simulink model "Linearize_Bare_Airframe"  (R2022a)
settings: Solver=VariableStepAuto  StartTime=0.0  StopTime=10.0  RelTol=1e-3
undefined symbols (not defined in the file): Aactuator, ac, AeroCoeff, EngineTable, F, fs, ft, g, hground, IC, kg, LandingGear, Light, m, MIL, s, Sensor, slug, state0, WMM2020
libraries: aerolibconvert2 x15, simulink x4, aerolibatmos2 x3, aerolibwind2 x3, sharedutil x3, aerolibbdyn x3, aerolibgravity2 x2, sharedtransform x1
(part 2 of 4)

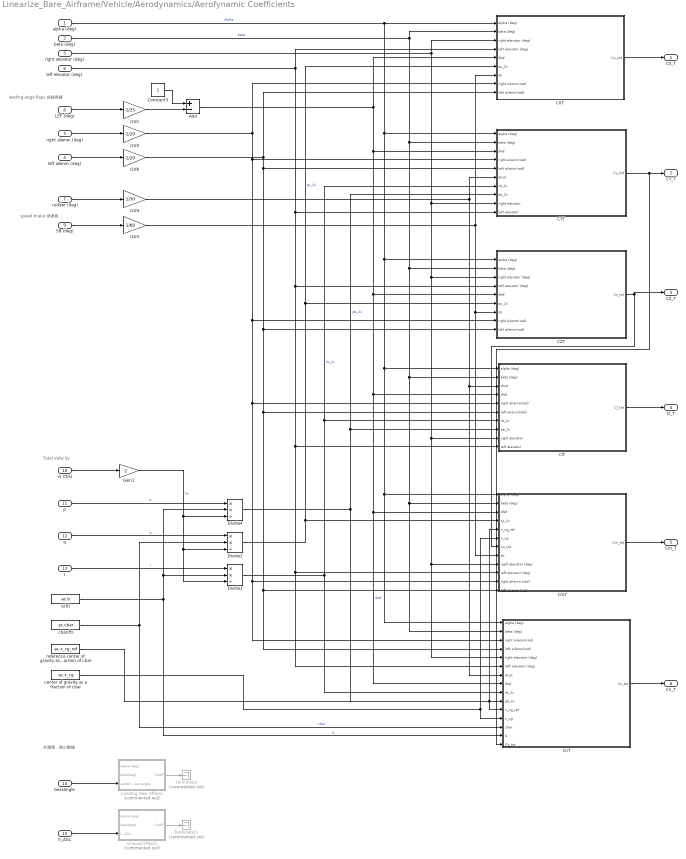
== system Linearize_Bare_Airframe/Vehicle/Aerodynamics/Aerofynamic Coefficients ==
  note: Total Velocity
  note: 未建模，缺少數據
  note: speed brake
      | 減速板
  note: leading-edge flaps
      | 前緣襟翼
  alpha (deg) : Inport
  beta (deg) : Inport  Port=2
  right alieron (deg) : Inport  Port=3
  left aileron (deg) : Inport  Port=4
  right elevator (deg) : Inport  Port=5
  left elevator (deg) : Inport  Port=6
  rudder (deg) : Inport  Port=7
  LEF (deg) : Inport  Port=8
  SB (deg) : Inport  Port=9
  vt (ft/s) : Inport  Port=10
  p : Inport  Port=11
  q : Inport  Port=12
  r : Inport  Port=13
  GearAngle : Inport  Port=14
  h_AGL : Inport  Port=15
  Add : Sum  Inputs=+-
  CXT : Subsystem
  CYT : Subsystem
  CZT : Subsystem
  ClT : Subsystem
  CmT : Subsystem
  CnT : Subsystem
  Constant3 : Constant
  Divide2 : Product  Inputs=**/
  Divide3 : Product  Inputs=**/
  Divide4 : Product  Inputs=**/
  Gain1 : Gain  Gain=2
  Ground Effects : Subsystem  Commented=on
  Landing Gear Effects : Subsystem  Commented=on
  Terminator : Terminator  Commented=on
  Terminator1 : Terminator  Commented=on
  b(ft) : Constant  Value=ac.b
  cbar(ft) : Constant  Value=ac.cbar
  center of gravity as a fraction of cbar : Constant  Value=ac.x_cg
  r2d1 : Gain  Gain=1/25  SaturateOnIntegerOverflow=on  OutDataTypeStr=Inherit: Same as input  ParamDataTypeStr=Inherit: Same as input
  r2d3 : Gain  Gain=1/60  SaturateOnIntegerOverflow=on  OutDataTypeStr=Inherit: Same as input  ParamDataTypeStr=Inherit: Same as input
  r2d4 : Gain  Gain=1/30  SaturateOnIntegerOverflow=on  OutDataTypeStr=Inherit: Same as input  ParamDataTypeStr=Inherit: Same as input
  r2d5 : Gain  Gain=1/20  SaturateOnIntegerOverflow=on  OutDataTypeStr=Inherit: Same as input  ParamDataTypeStr=Inherit: Same as input
  r2d6 : Gain  Gain=1/20  SaturateOnIntegerOverflow=on  OutDataTypeStr=Inherit: Same as input  ParamDataTypeStr=Inherit: Same as input
  reference center of gravity as a fraction of cbar : Constant  Value=ac.x_cg_ref
  CX_T : Outport  VectorParamsAs1DForOutWhenUnconnected=off
  CY_T : Outport  Port=2  VectorParamsAs1DForOutWhenUnconnected=off
  CZ_T : Outport  Port=3  VectorParamsAs1DForOutWhenUnconnected=off
  Cl_T : Outport  Port=4  VectorParamsAs1DForOutWhenUnconnected=off
  Cm_T : Outport  Port=5  VectorParamsAs1DForOutWhenUnconnected=off
  Cn_T : Outport  Port=6  VectorParamsAs1DForOutWhenUnconnected=off
  wires:
  alpha (deg)/1 -> CnT/1(alpha (deg)), CmT/1(alpha (deg)), ClT/1(alpha (deg)), CZT/1(alpha (deg)), CYT/1(alpha (deg)), CXT/1(alpha (deg))  "alpha"
  beta (deg)/1 -> CnT/2(beta (deg)), CmT/2(beta (deg)), ClT/2(beta (deg)), CZT/2(beta (deg)), CYT/2(beta (deg)), CXT/2("beta (deg) ")  "beta"
  right elevator (deg)/1 -> CmT/9(right elevator (deg)), CnT/5("right elevator (deg) "), ClT/9(right elevator), CZT/3(right elevator (deg)), CYT/9(right elevator), CXT/3(right elevator (deg))
  vt (ft/s)/1 -> Gain1/1
  q/1 -> Divide2/1  "q"
  r/1 -> Divide3/1  "r"
  Divide2/1 -> CXT/6(qc_2v), CZT/6(qc_2v), CmT/4(qc_2v)  "qc_2v"
  Divide3/1 -> CYT/7(rb_2v), ClT/7(rb_2v), CnT/9(rb_2v)  "rb_2v"
  Divide4/1 -> CYT/8(pb_2v), ClT/8(pb_2v), CnT/10(pb_2v)  "pb_2v"
  b(ft)/1 -> CnT/14(b), Divide3/2, Divide4/2  "b"
  cbar(ft)/1 -> CnT/13(cbar), Divide2/2  "cbar"
  reference center of gravity as a fraction of cbar/1 -> CmT/5(x_cg_ref), CnT/11(x_cg_ref)
  center of gravity as a fraction of cbar/1 -> CmT/6(x_cg), CnT/12(x_cg)
  CZT/1(Cz_tot) -> CZ_T/1, CmT/7(Cz_tot)
  CYT/1(Cy_tot) -> CnT/15(Cy_tot), CY_T/1
  CXT/1(Cx_tot) -> CX_T/1
  ClT/1(Cl_tot) -> Cl_T/1
  CmT/1(Cm_tot) -> Cm_T/1
  CnT/1(Cn_tot) -> Cn_T/1
  Add/1 -> CXT/5(dlef), CnT/8(dlef), CmT/3(dlef), ClT/4(dlef), CZT/5(dlef), CYT/3(dlef)  "dlef"
  rudder (deg)/1 -> r2d4/1
  SB (deg)/1 -> r2d3/1
  r2d1/1 -> Add/2
  Constant3/1 -> Add/1
  LEF (deg)/1 -> r2d1/1
  Gain1/1 -> Divide4/3, Divide3/3, Divide2/3  "2v"
  p/1 -> Divide4/1  "p"
  r2d3/1 -> CmT/8(sb), CZT/7(sb), CXT/7(sb)
  r2d4/1 -> CYT/6(drud), CnT/7(drud), ClT/3(drud)
  GearAngle/1 -> Landing Gear Effects/3(Landing Gear Angle)
  h_AGL/1 -> Ground Effects/3(h_AGL)
  Landing Gear Effects/1(Coeff) -> Terminator/1
  Ground Effects/1(Coeff) -> Terminator1/1
  left elevator (deg)/1 -> CZT/4(left elevator (deg)), CmT/10(left elevator (deg)), CnT/6(left elevator (deg)), ClT/10(left elevator), CYT/10(left elevator), CXT/4(left elevator (deg))
  right alieron (deg)/1 -> r2d5/1
  left aileron (deg)/1 -> r2d6/1
  r2d5/1 -> CmT/11(right aileron (rad)), CnT/3(right aileron(rad)), ClT/5(right aileron(rad)), CZT/8(right aileron(rad)), CYT/4(right aileron(rad)), CXT/8(right aileron(rad))
  r2d6/1 -> CXT/9(left aileron(rad)), CZT/9(left aileron(rad)), CmT/12(left aileron (rad)), CnT/4(left aileron(rad)), ClT/6(left aileron(rad)), CYT/5(left aileron(rad))

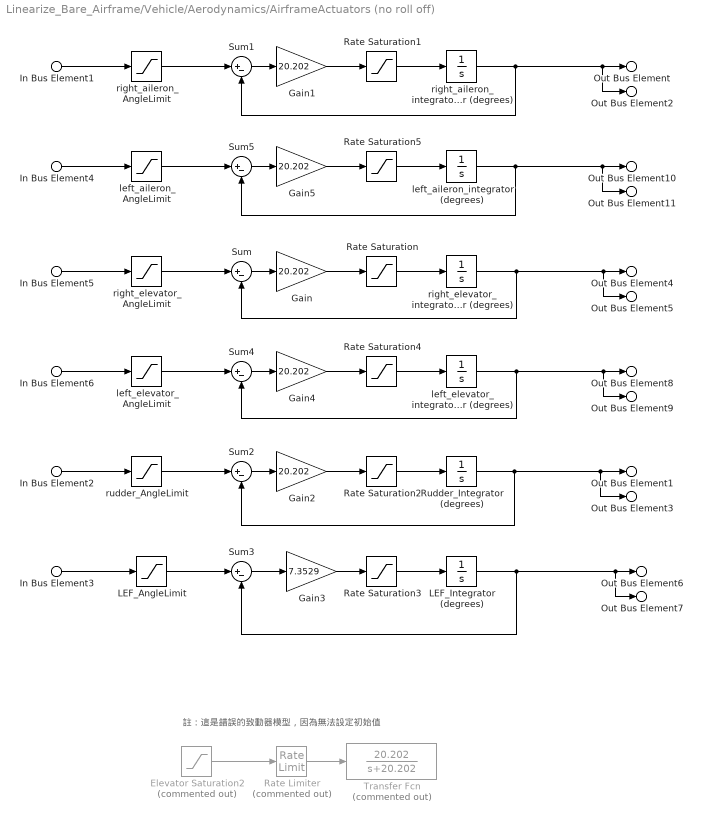
== system Linearize_Bare_Airframe/Vehicle/Aerodynamics/AirframeActuators (no roll off) ==
  note: 註：這是錯誤的致動器模型，因為無法設定初始值
  In Bus Element2 : Inport  PortName=fcs_cmd  Element=rudder
  In Bus Element3 : Inport  PortName=fcs_cmd  Element=LEF
  In Bus Element4 : Inport  PortName=fcs_cmd  Element=left aileron
  In Bus Element5 : Inport  PortName=fcs_cmd  Element=right elevator
  In Bus Element6 : Inport  PortName=fcs_cmd  Element=left elevator
  In Bus Element1 : Inport  PortName=fcs_cmd  Element=right aileron
  Elevator Saturation2 : Saturate  Commented=on  UpperLimit=25  LowerLimit=-25
  Gain{,1..2,4..5} (5 alike) : Gain  Gain=20.202  SaturateOnIntegerOverflow=on  OutDataTypeStr=Inherit: Same as input  ParamDataTypeStr=Inherit: Same as input
  Gain3 : Gain  Gain=7.3529  SaturateOnIntegerOverflow=on  OutDataTypeStr=Inherit: Same as input  ParamDataTypeStr=Inherit: Same as input
  LEF_AngleLimit : Saturate  UpperLimit=Aactuator.LEF.AngleLimitUpper  LowerLimit=Aactuator.LEF.AngleLimitLower
  LEF_Integrator (degrees) : Integrator  InitialCondition=Aactuator.LEF.IntegratorInitial  LimitOutput=on  UpperSaturationLimit=Aactuator.LEF.AngleLimitUpper  LowerSaturationLimit=Aactuator.LEF.AngleLimitLower
  Rate Saturation : Saturate  UpperLimit=Aactuator.right_elevator.RateLimitUpper  LowerLimit=Aactuator.right_elevator.RateLimitLower
  Rate Saturation1 : Saturate  UpperLimit=Aactuator.right_aileron.RateLimitUpper  LowerLimit=Aactuator.right_aileron.RateLimitLower
  Rate Saturation2 : Saturate  UpperLimit=Aactuator.rudder.RateLimitUpper  LowerLimit=Aactuator.rudder.RateLimitLower
  Rate Saturation3 : Saturate  UpperLimit=Aactuator.LEF.RateLimitUpper  LowerLimit=Aactuator.LEF.RateLimitLower
  Rate Saturation4 : Saturate  UpperLimit=Aactuator.left_elevator.RateLimitUpper  LowerLimit=Aactuator.left_elevator.RateLimitLower
  Rate Saturation5 : Saturate  UpperLimit=Aactuator.left_aileron.RateLimitUpper  LowerLimit=Aactuator.left_aileron.RateLimitLower
  Rate Limiter : RateLimiter  Commented=on  RisingSlewLimit=+60  FallingSlewLimit=-60  SampleTimeMode=inherited
  Rudder_Integrator (degrees) : Integrator  InitialCondition=Aactuator.rudder.IntegratorInitial  LimitOutput=on  UpperSaturationLimit=Aactuator.rudder.AngleLimitUpper  LowerSaturationLimit=Aactuator.rudder.AngleLimitLower
  Sum{,1..5} (6 alike) : Sum  Inputs=|+-  InputSameDT=on  SaturateOnIntegerOverflow=on  OutDataTypeStr=Inherit: Same as first input
  Transfer Fcn : TransferFcn  Commented=on  Numerator=[20.202]  Denominator=[1 20.202]
  left_aileron_AngleLimit : Saturate  UpperLimit=Aactuator.left_aileron.AngleLimitUpper  LowerLimit=Aactuator.left_aileron.AngleLimitLower
  left_aileron_integrator (degrees) : Integrator  InitialCondition=Aactuator.left_aileron.IntegratorInitial  LimitOutput=on  UpperSaturationLimit=Aactuator.left_aileron.AngleLimitUpper  LowerSaturationLimit=Aactuator.left_aileron.AngleLimitLower
  left_elevator_AngleLimit : Saturate  UpperLimit=Aactuator.left_elevator.AngleLimitUpper  LowerLimit=Aactuator.left_elevator.AngleLimitLower
  left_elevator_integrator (degrees) : Integrator  InitialCondition=Aactuator.left_elevator.IntegratorInitial  LimitOutput=on  UpperSaturationLimit=Aactuator.left_elevator.AngleLimitUpper  LowerSaturationLimit=Aactuator.left_elevator.AngleLimitLower
  right_aileron_AngleLimit : Saturate  UpperLimit=Aactuator.right_aileron.AngleLimitUpper  LowerLimit=Aactuator.right_aileron.AngleLimitLower
  right_aileron_integrator (degrees) : Integrator  InitialCondition=Aactuator.right_aileron.IntegratorInitial  LimitOutput=on  UpperSaturationLimit=Aactuator.right_aileron.AngleLimitUpper  LowerSaturationLimit=Aactuator.right_aileron.AngleLimitLower
  right_elevator_AngleLimit : Saturate  UpperLimit=Aactuator.right_elevator.AngleLimitUpper  LowerLimit=Aactuator.right_elevator.AngleLimitLower  LinearizeAsGain=off
  right_elevator_integrator (degrees) : Integrator  InitialCondition=Aactuator.right_elevator.IntegratorInitial  LimitOutput=on  UpperSaturationLimit=Aactuator.right_elevator.AngleLimitUpper  LowerSaturationLimit=Aactuator.right_elevator.AngleLimitLower
  rudder_AngleLimit : Saturate  UpperLimit=Aactuator.rudder.AngleLimitUpper  LowerLimit=Aactuator.rudder.AngleLimitLower
  Out Bus Element : Outport  PortName=ActPositions  Element=right Aileron_deg
  Out Bus Element1 : Outport  PortName=ActPositions  Element=Rudder_deg
  Out Bus Element4 : Outport  PortName=ActPositions  Element=right Elevator_deg
  Out Bus Element6 : Outport  PortName=ActPositions  Element=LEF_deg
  Out Bus Element8 : Outport  PortName=ActPositions  Element=left Elevator_deg
  Out Bus Element10 : Outport  PortName=ActPositions  Element=left Aileron_deg
  Out Bus Element2 : Outport  Port=2  PortName=ActSensor_Out  Element=right Aileron_deg
  Out Bus Element3 : Outport  Port=2  PortName=ActSensor_Out  Element=Rudder_deg
  Out Bus Element5 : Outport  Port=2  PortName=ActSensor_Out  Element=right Elevator_deg
  Out Bus Element7 : Outport  Port=2  PortName=ActSensor_Out  Element=LEF_deg
  Out Bus Element9 : Outport  Port=2  PortName=ActSensor_Out  Element=left Elevator_deg
  Out Bus Element11 : Outport  Port=2  PortName=ActSensor_Out  Element=left Aileron_deg
  wires:
  Gain/1 -> Rate Saturation/1
  Gain1/1 -> Rate Saturation1/1
  In Bus Element5/1 -> right_elevator_AngleLimit/1
  Rate Saturation/1 -> right_elevator_integrator (degrees)/1
  right_aileron_integrator (degrees)/1 -> Out Bus Element2/1, Out Bus Element/1, Sum1/2
  Rate Saturation1/1 -> right_aileron_integrator (degrees)/1
  Gain2/1 -> Rate Saturation2/1
  Sum1/1 -> Gain1/1
  Rudder_Integrator (degrees)/1 -> Out Bus Element3/1, Out Bus Element1/1, Sum2/2
  Rate Saturation2/1 -> Rudder_Integrator (degrees)/1
  Sum/1 -> Gain/1
  Sum2/1 -> Gain2/1
  right_elevator_integrator (degrees)/1 -> Sum/2, Out Bus Element5/1, Out Bus Element4/1
  In Bus Element1/1 -> right_aileron_AngleLimit/1
  In Bus Element2/1 -> rudder_AngleLimit/1
  LEF_Integrator (degrees)/1 -> Out Bus Element6/1, Out Bus Element7/1, Sum3/2
  In Bus Element3/1 -> LEF_AngleLimit/1
  Sum3/1 -> Gain3/1
  Rate Saturation3/1 -> LEF_Integrator (degrees)/1
  Gain3/1 -> Rate Saturation3/1
  Sum4/1 -> Gain4/1
  Gain4/1 -> Rate Saturation4/1
  Rate Saturation4/1 -> left_elevator_integrator (degrees)/1
  In Bus Element6/1 -> left_elevator_AngleLimit/1
  left_elevator_integrator (degrees)/1 -> Sum4/2, Out Bus Element9/1, Out Bus Element8/1
  Gain5/1 -> Rate Saturation5/1
  Rate Saturation5/1 -> left_aileron_integrator (degrees)/1
  Sum5/1 -> Gain5/1
  left_aileron_integrator (degrees)/1 -> Out Bus Element11/1, Out Bus Element10/1, Sum5/2
  In Bus Element4/1 -> left_aileron_AngleLimit/1
  right_aileron_AngleLimit/1 -> Sum1/1
  left_aileron_AngleLimit/1 -> Sum5/1
  left_elevator_AngleLimit/1 -> Sum4/1
  right_elevator_AngleLimit/1 -> Sum/1
  rudder_AngleLimit/1 -> Sum2/1
  LEF_AngleLimit/1 -> Sum3/1
  Rate Limiter/1 -> Transfer Fcn/1
  Elevator Saturation2/1 -> Rate Limiter/1

== system Linearize_Bare_Airframe/Vehicle/Aerodynamics/Leading Edge Flap ==
  note: $\delta_{LEF} =1.38\frac{2s+7.25}{s+7.25}\alpha -9.05\frac{\bar{q} }{p_s }+1.45$
      | $\alpha$ 的單位：deg
      | $\bar{q}$ 是動壓， $p_s$ 是靜壓，兩者單位要一致 (公制：1Pa = 1 $N/m^2$ = 1 $\mathrm{kg}/\left(m{\cdot s}^2 \right)$ ；英制：1psf = 1 $\mathrm{lbf}/{\mathrm{ft}}^2$ = 1 $\mathrm{slugs}/\left(\mathrm{ft}\cdot s^2 \right)$ )
  vt (m/s) : Inport
  rho (kg/m^3) : Inport  Port=2
  P (Pa) : Inport  Port=3
  alpha (deg) : Inport  Port=4
  Divide1 : Product  Inputs=*/
  Divide2 : Product  Inputs=**
  Gain2 : Gain  Gain=1.38  SaturateOnIntegerOverflow=on  OutDataTypeStr=Inherit: Same as input  ParamDataTypeStr=Inherit: Same as input
  LEF Rate Limiter : RateLimiter  RisingSlewLimit=Aactuator.LEF.RateLimitUpper  FallingSlewLimit=Aactuator.LEF.RateLimitLower  SampleTimeMode=inherited  InitialCondition=Aactuator.LEF.IntegratorInitial
  LEF Saturation : Saturate  UpperLimit=Aactuator.LEF.AngleLimitUpper  LowerLimit=Aactuator.LEF.AngleLimitLower
  Square1 : Math  Operator=square  SignedPower=on
  Sum : Sum  Inputs=-|+|+  InputSameDT=on  SaturateOnIntegerOverflow=on  OutDataTypeStr=Inherit: Same as first input
  Transfer Fcn : TransferFcn  Numerator=[2 7.25]  Denominator=[1 7.25]
  coeff1 : Constant  Value=1.45
  r2d2 : Gain  Gain=0.5  SaturateOnIntegerOverflow=on  OutDataTypeStr=Inherit: Same as input  ParamDataTypeStr=Inherit: Same as input
  r2d6 : Gain  Gain=9.05  SaturateOnIntegerOverflow=on  OutDataTypeStr=Inherit: Same as input  ParamDataTypeStr=Inherit: Same as input
  Out Bus Element3 : Outport  PortName=ActSensor_Out  Element=LEF_deg
  Out Bus Element2 : Outport  Port=2  PortName=ActPositions  Element=LEF_deg
  wires:
  Transfer Fcn/1 -> Gain2/1
  coeff1/1 -> Sum/3
  r2d6/1 -> Sum/1
  Square1/1 -> Divide2/1
  alpha (deg)/1 -> Transfer Fcn/1  "alpha (deg)"
  P (Pa)/1 -> Divide1/2
  vt (m/s)/1 -> Square1/1
  rho (kg/m^3)/1 -> Divide2/2  "rho(kg/m^3)"
  Divide1/1 -> r2d6/1
  Sum/1 -> LEF Saturation/1
  LEF Saturation/1 -> LEF Rate Limiter/1
  Divide2/1 -> r2d2/1
  r2d2/1 -> Divide1/1  "qbar (Pa)"
  Gain2/1 -> Sum/2
  LEF Rate Limiter/1 -> Out Bus Element2/1, Out Bus Element3/1

== system Linearize_Bare_Airframe/Vehicle/LandingGear GroundReaction/L Main Gear Geometry Forces and Moments ==
  note: $z_c^E$
  note: $z_g^E$
  note: 飛機重心在慣性座標的高度
  note: 詹庭宇:
      | 此起落架模組源自MATLAB Simulink Example:HL-20
      | 我有做正負號的訂正
  note: 詹庭宇:
      | 此起落架模組源自MATLAB Simulink Example:HL-20
      | 我有做正負號的訂正
  note: 定義：
      | 慣性座標+Z軸朝下
      | 體座標+Z軸朝下
  note: $z_g^E =z_c^E +C_{31} {\left(x_g^b -x_c^b \right)}+C_{32} {\left(y_g^b -y_c^b \right)}+C_{33} {\left(z_g^b -z_c^b \right)}$
  note: $z_r^E$
  note: 體座標轉至慣性座標的旋轉矩陣
  note: 體座標轉至慣性座標的旋轉矩陣
  note: 詹庭宇:拿掉/忽略輪胎側向力模型，Fy=0
  ground_z_ft : Inport
  plant : Inport  Port=2
  GearLoc : Inport  Port=3
  Bus Selector3 : BusSelector  OutputSignals=altitude,DCM_eb,DCM_be
  Calc Gear Force and Pos : Subsystem
  GenerateGroundFM : Subsystem
  Rotate pos to earth axes : Product  Multiplication=Matrix(*)  InputSameDT=on  SaturateOnIntegerOverflow=on  OutDataTypeStr=Inherit: Same as first input
  Sum3 : Sum
  Zg : Selector  InputPortWidth=3  IndexOptions=Index vector (dialog)  Indices=3  OutputSizes=1
  detect_WOW : RelationalOperator  OutDataTypeStr=boolean  InputSameDT=off
  FM : Outport
  WOW : Outport  Port=2
  GearCmprs : Outport  Port=3
  wires:
  Rotate pos to earth axes/1 -> Zg/1
  Bus Selector3/1 -> [ZcL], [Xe]  "<altitude>"
  detect_WOW/1 -> GenerateGroundFM/Enable, WOW/1, Calc Gear Force and Pos/1(WOW)
  Bus Selector3/2 -> [DCM_eb]  "<DCM_eb>"
  Zg/1 -> Sum3/2
  Sum3/1 -> detect_WOW/1
  Calc Gear Force and Pos/3(ZgB_prime) -> GenerateGroundFM/3(ZgB_prime)
  GearLoc/1 -> Calc Gear Force and Pos/3(Xg), Rotate pos to earth axes/2, GenerateGroundFM/1(GearLoc)
  Calc Gear Force and Pos/1(dZ_strut) -> GearCmprs/1
  [DCM_eb] -> Calc Gear Force and Pos/5(DCM_eb)
  GenerateGroundFM/1(FM) -> FM/1
  [Xe] -> Sum3/1
  [DCM_eb] -> Rotate pos to earth axes/1
  Calc Gear Force and Pos/2(Fn_strut) -> GenerateGroundFM/2(Fn_strut)
  plant/1 -> Bus Selector3/1, GenerateGroundFM/5(plant)
  ground_z_ft/1 -> detect_WOW/2, Calc Gear Force and Pos/2(ZrL)
  Bus Selector3/3 -> GenerateGroundFM/4(DCM_be)  "<DCM_be>"
  [ZcL] -> Calc Gear Force and Pos/4(ZcL)

== system Linearize_Bare_Airframe/Vehicle/LandingGear GroundReaction/Nose Gear Geometry Forces and Moments ==
  note: $z_c^E$
  note: $z_g^E$
  note: 飛機重心在慣性座標的高度
  note: 詹庭宇:
      | 此起落架模組源自MATLAB Simulink Example:HL-20
      | 我有做正負號的訂正
  note: 詹庭宇:
      | 此起落架模組源自MATLAB Simulink Example:HL-20
      | 我有做正負號的訂正
  note: 定義：
      | 慣性座標+Z軸朝下
      | 體座標+Z軸朝下
  note: $z_g^E =z_c^E +C_{31} {\left(x_g^b -x_c^b \right)}+C_{32} {\left(y_g^b -y_c^b \right)}+C_{33} {\left(z_g^b -z_c^b \right)}$
  note: $z_r^E$
  note: 體座標轉至慣性座標的旋轉矩陣
  note: 體座標轉至慣性座標的旋轉矩陣
  note: 詹庭宇:拿掉/忽略輪胎側向力模型，Fy=0
  ground_z_ft : Inport
  plant : Inport  Port=2
  GearLoc : Inport  Port=3
  Bus Selector3 : BusSelector  OutputSignals=altitude,DCM_eb,DCM_be
  Calc Gear Force and Pos : Subsystem
  GenerateGroundFM : Subsystem
  Rotate pos to earth axes : Product  Multiplication=Matrix(*)  InputSameDT=on  SaturateOnIntegerOverflow=on  OutDataTypeStr=Inherit: Same as first input
  Sum3 : Sum
  Zg : Selector  InputPortWidth=3  IndexOptions=Index vector (dialog)  Indices=3  OutputSizes=1
  detect_WOW : RelationalOperator  OutDataTypeStr=boolean  InputSameDT=off
  FM : Outport
  WOW : Outport  Port=2
  GearCmprs : Outport  Port=3
  wires:
  Rotate pos to earth axes/1 -> Zg/1
  Bus Selector3/1 -> [ZcL], [Xe]  "<altitude>"
  detect_WOW/1 -> GenerateGroundFM/Enable, WOW/1, Calc Gear Force and Pos/1(WOW)
  Zg/1 -> Sum3/2
  Sum3/1 -> detect_WOW/1
  Calc Gear Force and Pos/3(ZgB_prime) -> GenerateGroundFM/3(ZgB_prime)
  GearLoc/1 -> GenerateGroundFM/1(GearLoc), Calc Gear Force and Pos/3(Xg), Rotate pos to earth axes/2
  Calc Gear Force and Pos/1(dZ_strut) -> GearCmprs/1
  [DCM_eb] -> Calc Gear Force and Pos/5(DCM_eb)
  GenerateGroundFM/1(FM) -> FM/1
  [Xe] -> Sum3/1
  [DCM_eb] -> Rotate pos to earth axes/1
  Calc Gear Force and Pos/2(Fn_strut) -> GenerateGroundFM/2(Fn_strut)
  plant/1 -> Bus Selector3/1, GenerateGroundFM/5(plant)
  ground_z_ft/1 -> detect_WOW/2, Calc Gear Force and Pos/2(ZrL)
  [ZcL] -> Calc Gear Force and Pos/4(ZcL)
  Bus Selector3/2 -> [DCM_eb]  "<DCM_eb>"
  Bus Selector3/3 -> GenerateGroundFM/4(DCM_be)  "<DCM_be>"

== system Linearize_Bare_Airframe/Vehicle/LandingGear GroundReaction/R Main Gear Geometry Forces and Moments ==
  note: $z_c^E$
  note: $z_g^E$
  note: 飛機重心在慣性座標的高度
  note: 詹庭宇:
      | 此起落架模組源自MATLAB Simulink Example:HL-20
      | 我有做正負號的訂正
  note: 詹庭宇:
      | 此起落架模組源自MATLAB Simulink Example:HL-20
      | 我有做正負號的訂正
  note: 定義：
      | 慣性座標+Z軸朝下
      | 體座標+Z軸朝下
  note: $z_g^E =z_c^E +C_{31} {\left(x_g^b -x_c^b \right)}+C_{32} {\left(y_g^b -y_c^b \right)}+C_{33} {\left(z_g^b -z_c^b \right)}$
  note: $z_r^E$
  note: 體座標轉至慣性座標的旋轉矩陣
  note: 體座標轉至慣性座標的旋轉矩陣
  note: 詹庭宇:拿掉/忽略輪胎側向力模型，Fy=0
  ground_z_ft : Inport
  plant : Inport  Port=2
  GearLoc : Inport  Port=3
  Bus Selector3 : BusSelector  OutputSignals=altitude,DCM_eb,DCM_be
  Calc Gear Force and Pos : Subsystem
  GenerateGroundFM : Subsystem
  Rotate pos to earth axes : Product  Multiplication=Matrix(*)  InputSameDT=on  SaturateOnIntegerOverflow=on  OutDataTypeStr=Inherit: Same as first input
  Sum3 : Sum
  Zg : Selector  InputPortWidth=3  IndexOptions=Index vector (dialog)  Indices=3  OutputSizes=1
  detect_WOW : RelationalOperator  OutDataTypeStr=boolean  InputSameDT=off
  FM : Outport
  WOW : Outport  Port=2
  GearCmprs : Outport  Port=3
  wires:
  Rotate pos to earth axes/1 -> Zg/1
  Bus Selector3/1 -> [ZcL], [Xe]  "<altitude>"
  detect_WOW/1 -> Calc Gear Force and Pos/1(WOW), GenerateGroundFM/Enable, WOW/1
  Zg/1 -> Sum3/2
  Sum3/1 -> detect_WOW/1
  Calc Gear Force and Pos/3(ZgB_prime) -> GenerateGroundFM/3(ZgB_prime)
  GearLoc/1 -> Rotate pos to earth axes/2, GenerateGroundFM/1(GearLoc), Calc Gear Force and Pos/3(Xg)
  Calc Gear Force and Pos/1(dZ_strut) -> GearCmprs/1
  [DCM_eb] -> Calc Gear Force and Pos/5(DCM_eb)
  GenerateGroundFM/1(FM) -> FM/1
  [Xe] -> Sum3/1
  [DCM_eb] -> Rotate pos to earth axes/1
  Calc Gear Force and Pos/2(Fn_strut) -> GenerateGroundFM/2(Fn_strut)
  plant/1 -> GenerateGroundFM/5(plant), Bus Selector3/1
  ground_z_ft/1 -> detect_WOW/2, Calc Gear Force and Pos/2(ZrL)
  [ZcL] -> Calc Gear Force and Pos/4(ZcL)
  Bus Selector3/2 -> [DCM_eb]  "<DCM_eb>"
  Bus Selector3/3 -> GenerateGroundFM/4(DCM_be)  "<DCM_be>"

== system Linearize_Bare_Airframe/Vehicle/Propulsion/Actuators ==
  In Bus Element : Inport  PortName=Commands  Element=TVC_rY
  In Bus Element4 : Inport  PortName=Commands  Element=TVC_lY
  In Bus Element1 : Inport  PortName=Commands  Element=TVC_rZ
  In Bus Element2 : Inport  PortName=Commands  Element=TVC_lZ
  Gain{1..2,4..5} (4 alike) : Gain  Gain=20.202  SaturateOnIntegerOverflow=on  OutDataTypeStr=Inherit: Same as input  ParamDataTypeStr=Inherit: Same as input
  Rate Saturation1 : Saturate  UpperLimit=Aactuator.TVC_Y.RateLimitUpper  LowerLimit=Aactuator.TVC_Y.RateLimitLower
  Rate Saturation2 : Saturate  UpperLimit=Aactuator.TVC_Z.RateLimitUpper  LowerLimit=Aactuator.TVC_Z.RateLimitLower
  Rate Saturation4 : Saturate  UpperLimit=Aactuator.TVC_Y.RateLimitUpper  LowerLimit=Aactuator.TVC_Y.RateLimitLower
  Rate Saturation5 : Saturate  UpperLimit=Aactuator.TVC_Z.RateLimitUpper  LowerLimit=Aactuator.TVC_Z.RateLimitLower
  Sum{1..2,4..5} (4 alike) : Sum  Inputs=|+-  InputSameDT=on  SaturateOnIntegerOverflow=on  OutDataTypeStr=Inherit: Same as first input
  TVC_lY Saturation : Saturate  UpperLimit=Aactuator.TVC_Z.AngleLimitUpper  LowerLimit=Aactuator.TVC_Z.AngleLimitLower
  TVC_lY_Integrator (degrees) : Integrator  InitialCondition=Aactuator.TVC_Y.IntegratorInitial  LimitOutput=on  UpperSaturationLimit=Aactuator.TVC_Y.AngleLimitUpper  LowerSaturationLimit=Aactuator.TVC_Y.AngleLimitLower
  TVC_lZ Saturation : Saturate  UpperLimit=Aactuator.TVC_Y.AngleLimitUpper  LowerLimit=Aactuator.TVC_Y.AngleLimitLower
  TVC_lZ_Integrator (degrees) : Integrator  InitialCondition=Aactuator.TVC_Z.IntegratorInitial  LimitOutput=on  UpperSaturationLimit=Aactuator.TVC_Z.AngleLimitUpper  LowerSaturationLimit=Aactuator.TVC_Z.AngleLimitLower
  TVC_rY Saturation : Saturate  UpperLimit=Aactuator.TVC_Z.AngleLimitUpper  LowerLimit=Aactuator.TVC_Z.AngleLimitLower
  TVC_rY_Integrator (degrees) : Integrator  InitialCondition=Aactuator.TVC_Y.IntegratorInitial  LimitOutput=on  UpperSaturationLimit=Aactuator.TVC_Y.AngleLimitUpper  LowerSaturationLimit=Aactuator.TVC_Y.AngleLimitLower
  TVC_rZ Saturation : Saturate  UpperLimit=Aactuator.TVC_Y.AngleLimitUpper  LowerLimit=Aactuator.TVC_Y.AngleLimitLower
  TVC_rZ_Integrator (degrees) : Integrator  InitialCondition=Aactuator.TVC_Z.IntegratorInitial  LimitOutput=on  UpperSaturationLimit=Aactuator.TVC_Z.AngleLimitUpper  LowerSaturationLimit=Aactuator.TVC_Z.AngleLimitLower
  Out Bus Element : Outport  PortName=ActPositions  Element=TVC_rY_pitch_deg
  Out Bus Element1 : Outport  PortName=ActPositions  Element=TVC_rZ_yaw_deg
  Out Bus Element4 : Outport  PortName=ActPositions  Element=TVC_lY_pitch_deg
  Out Bus Element5 : Outport  PortName=ActPositions  Element=TVC_lZ_yaw_deg
  Out Bus Element2 : Outport  Port=2  PortName=ActSensor_Out  Element=TVC_rY_pitch_deg
  Out Bus Element3 : Outport  Port=2  PortName=ActSensor_Out  Element=TVC_rZ_yaw_deg
  Out Bus Element6 : Outport  Port=2  PortName=ActSensor_Out  Element=TVC_lY_pitch_deg
  Out Bus Element7 : Outport  Port=2  PortName=ActSensor_Out  Element=TVC_lZ_yaw_deg
  wires:
  Sum5/1 -> Gain5/1
  TVC_rY_Integrator (degrees)/1 -> Out Bus Element2/1, Out Bus Element/1, Sum4/2  "TVC_rY_pitch_deg"
  Sum4/1 -> Gain4/1
  In Bus Element1/1 -> TVC_rY Saturation/1  "Commands_TVC_rZ_yaw_deg"
  TVC_rZ_Integrator (degrees)/1 -> Out Bus Element3/1, Out Bus Element1/1, Sum5/2  "TVC_rZ_yaw_deg"
  In Bus Element/1 -> TVC_rZ Saturation/1  "Commands_TVC_rY_pitch_deg"
  Rate Saturation5/1 -> TVC_rZ_Integrator (degrees)/1
  Gain4/1 -> Rate Saturation4/1
  Gain5/1 -> Rate Saturation5/1
  Rate Saturation4/1 -> TVC_rY_Integrator (degrees)/1
  TVC_lZ_Integrator (degrees)/1 -> Out Bus Element7/1, Out Bus Element5/1, Sum2/2  "TVC_lZ_yaw_deg"
  Gain1/1 -> Rate Saturation1/1
  Gain2/1 -> Rate Saturation2/1
  Rate Saturation1/1 -> TVC_lY_Integrator (degrees)/1
  Rate Saturation2/1 -> TVC_lZ_Integrator (degrees)/1
  Sum1/1 -> Gain1/1
  In Bus Element2/1 -> TVC_lY Saturation/1  "Commands_TVC_lZ_yaw_deg"
  Sum2/1 -> Gain2/1
  In Bus Element4/1 -> TVC_lZ Saturation/1  "Commands_TVC_lY_pitch_deg"
  TVC_lY_Integrator (degrees)/1 -> Out Bus Element6/1, Out Bus Element4/1, Sum1/2  "TVC_lY_pitch_deg"
  TVC_rZ Saturation/1 -> Sum4/1  "TVC_rY"
  TVC_rY Saturation/1 -> Sum5/1  "TVC_rZ"
  TVC_lZ Saturation/1 -> Sum1/1  "TVC_lY"
  TVC_lY Saturation/1 -> Sum2/1  "TVC_lZ"

== system Linearize_Bare_Airframe/Vehicle/Propulsion/Afterburning Turbofan Jet Engine ==
  note: TODO: 發動機模型不完整，要看參考文獻進行更完整建模
  note: 參考文獻： Nguyen, T. Luat, et al., "Simulator Study of StallPost-Stall Characteristics of a Fighter Airplane with Relaxed Longitudinal Static Stability," NASA Technical Paper 1538 , Dec. 1979.
  note: $pow{\left(\delta_{th} \right)}={\left\{\begin{array}{c} 64.94\delta_{th} \ ,\\ 217.38\delta_{th} -117.38\ ,\ \ \ \end{array}\begin{array}{c} if{\mathrm{\ }\delta }_{th} \le 0.77\\ if{\mathrm{\ }\delta }_{th} >0.77 \end{array}\right)}$
  note: $T={\left\{\begin{array}{c} T_{idle} +{\left(T_{mil} -T_{idle} \right)}{\left(\frac{pow}{50}\right)},\ \ \ \ \ \ \ \ if\ pow<50\\ T_{mil} +{\left(T_{max} -T_{mil} \right)}{\left(\frac{pow-50}{50}\right)},\ \ \ if\ pow\ge 50 \end{array}\begin{array}{c} \ \\ \ \ \end{array}\right)}$
  note: 功率位準 power level
  note: 油門推桿位置 $0\le \delta_{th} \le 1$
  Mach : Inport
  H (ft) : Inport  Port=2
  Tc (lbf) : Inport  Port=3
  Add : Sum  Inputs=+-
  Add1 : Sum
  Add2 : Sum
  Constant : Constant
  Constant1 : Constant  Value=0
  Gain : Gain  Gain=64.94
  Gain1 : Gain  Gain=217.38
  If : If  IfExpression=u1<50  ElseIfExpressions=u1>=50  ShowElse=off
  If Action Subsystem : Subsystem  TreatAsAtomicUnit=on
  If Action Subsystem1 : Subsystem  TreatAsAtomicUnit=on
  If Action Subsystem2 : Subsystem  TreatAsAtomicUnit=on
  If Action Subsystem3 : Subsystem  TreatAsAtomicUnit=on
  If Action Subsystem4 : Subsystem  TreatAsAtomicUnit=on
  If Action Subsystem5 : Subsystem  TreatAsAtomicUnit=on
  If Action Subsystem6 : Subsystem  TreatAsAtomicUnit=on
  If1 : If  IfExpression=u1<50  ElseIfExpressions=u1>=50  ShowElse=off
  If2 : If  NumInputs=3  IfExpression=u3 == u1  ElseIfExpressions=u3>u1 & u3<=u2
  Merge : Merge  Inputs=3
  Mux : Mux  Inputs=2
  Mux1 : Mux  Inputs=2
  Mux4 : Mux  Inputs=5
  Saturation Dynamic : simulink/Discontinuities/Saturation Dynamic  OutMin=[]  OutMax=[]  OutDataTypeStr=Inherit: Same as second input  OutDataType=fixdt(1, 16)  OutScaling=2^-10  DoSatur=off
  Thrust Tidle : Interpolation_n-D  Table=EngineTable.idle  InternalRulePriority=Speed
  Thrust Tmax : Interpolation_n-D  Table=EngineTable.maximum  InternalRulePriority=Speed
  Thrust Tmil : Interpolation_n-D  Table=EngineTable.military  InternalRulePriority=Speed
  To Workspace : ToWorkspace  VariableName=T_max_min  SaveFormat=Timeseries  SampleTime=-1
  To Workspace1 : ToWorkspace  VariableName=check_engine  SaveFormat=Timeseries  SampleTime=-1
  To Workspace2 : ToWorkspace  VariableName=Mach_alt_input  SaveFormat=Timeseries  SampleTime=-1
  afterburner_off : Constant  Value=2
  afterburner_on : Constant  Value=3
  attitude Prelookup : PreLookup  BreakpointsData=EngineTable.attitude_Prelookup  IndexSearchMethod=Linear search  BeginIndexSearchUsingPreviousIndexResult=on  DiagnosticForOutOfRangeInput=Warning
  constant : Constant  Value=117.38
  idle : Constant
  mach Prelookup : PreLookup  BreakpointsData=EngineTable.mach_Prelookup  IndexSearchMethod=Linear search  BeginIndexSearchUsingPreviousIndexResult=on  DiagnosticForOutOfRangeInput=Warning
  T (lbf) : Outport  VectorParamsAs1DForOutWhenUnconnected=off
  engine_state : Outport  Port=2  VectorParamsAs1DForOutWhenUnconnected=off
  wires:
  Mach/1 -> mach Prelookup/1, Mux/2
  H (ft)/1 -> attitude Prelookup/1, Mux/1
  Add2/1 -> Saturation Dynamic/3, Mux1/2  "T_min"
  Add1/1 -> Saturation Dynamic/1, Mux1/1  "T_max"
  attitude Prelookup/2 -> Thrust Tmil/4, Thrust Tmax/4, Thrust Tidle/4
  Mux1/1 -> To Workspace/1
  Mux/1 -> To Workspace2/1
  Gain1/1 -> Add/1
  If Action Subsystem1/1(T_max1) -> Add1/2
  Constant/1 -> Gain1/1
  mach Prelookup/1 -> Thrust Tmil/1, Thrust Tmax/1, Thrust Tidle/1
  If/2 -> If Action Subsystem1/Action
  If1/2 -> If Action Subsystem3/Action
  If Action Subsystem3/1(T_min) -> Add2/2
  If Action Subsystem2/1(T_min) -> Add2/1
  If1/1 -> If Action Subsystem2/Action
  Gain/1 -> Mux4/2, If1/1  "pow"
  If Action Subsystem/1(T_max1) -> Add1/1
  mach Prelookup/2 -> Thrust Tmil/2, Thrust Tmax/2, Thrust Tidle/2
  Thrust Tidle/1 -> Mux4/3, If2/1  "Tidle"
  If/1 -> If Action Subsystem/Action
  Add/1 -> Mux4/1, If/1  "pow"
  constant/1 -> Add/2
  Mux4/1 -> If Action Subsystem1/1("input "), If Action Subsystem2/1("input "), If Action Subsystem3/1("input "), To Workspace1/1, If Action Subsystem/1("input ")
  Constant1/1 -> Gain/1
  attitude Prelookup/1 -> Thrust Tmil/3, Thrust Tmax/3, Thrust Tidle/3
  If2/1 -> If Action Subsystem4/Action
  If2/3 -> If Action Subsystem6/Action
  idle/1 -> If Action Subsystem4/1(In1)
  afterburner_on/1 -> If Action Subsystem6/1(In1)
  Thrust Tmil/1 -> If2/2, Mux4/4  "Tmil"
  Thrust Tmax/1 -> Mux4/5
  If Action Subsystem6/1(Out1) -> Merge/3
  If Action Subsystem5/1(Out1) -> Merge/2
  If Action Subsystem4/1(Out1) -> Merge/1
  afterburner_off/1 -> If Action Subsystem5/1(In1)
  If2/2 -> If Action Subsystem5/Action
  Saturation Dynamic/1 -> T (lbf)/1, If2/3  "Thrust (lbf)"
  Merge/1 -> engine_state/1
  Tc (lbf)/1 -> Saturation Dynamic/2

== system Linearize_Bare_Airframe/Vehicle/Propulsion/Thrust Vector Nozzle ZY1 ==
  note: ${\left[\begin{array}{c} F_x^{{\left(T\right)}} \\ F_y^{{\left(T\right)}} \\ F_z^{{\left(T\right)}} \end{array}\right]}={\left[\begin{array}{c} T_x \\ T_y \\ T_z \end{array}\right]}={\left[\begin{array}{c} T_{lx} \\ T_{ly} \\ T_{lz} \end{array}\right]}+{\left[\begin{array}{c} T_{rx} \\ T_{ry} \\ T_{rz} \end{array}\right]}=\frac{T}{2}{\left[\begin{array}{cc} & \cos \delta_{lz} \cos \delta_{ly} +\mathrm{cos}\delta_{rz} \cos \delta_{ry} \\ & \sin \delta_{lz} +\sin \delta_{rz} \\ - & \cos \delta_{lz} \sin \delta_{ly} -\cos \delta_{rz} \sin \delta_{ry} \end{array}\right]}$
  note: ${\left[\begin{array}{c} M_x^{{\left(T\right)}} \\ M_y^{{\left(T\right)}} \\ M_z^{{\left(T\right)}} \end{array}\right]}={\left[\begin{array}{c} M_{lx} \\ M_{ly} \\ M_{lz} \end{array}\right]}+{\left[\begin{array}{c} M_{rx} \\ M_{ry} \\ M_{rz} \end{array}\right]}=\frac{T}{2}{\left[\begin{array}{l} m_T \cos \delta_{lz} \sin \delta_{ly} -m_T \mathrm{cos}\delta_{rz} \sin \delta_{ry} \\ -l_T \cos \delta_{lz} \sin \delta_{ly} -l_T \mathrm{cos}\delta_{rz} \sin \delta_{ry} \\ {-l}_T \sin \delta_{lz} -l_T \sin \delta_{rz} \end{array}\right]}$
  note: 單一噴嘴的推力
  T1 : Inport
  Actuator (deg) : Inport  Port=2
  " lt1" : Inport  Port=3
  " mt" : Inport  Port=4
  Add{,1..2,4} (4 alike) : Sum
  Add3 : Sum  Inputs=+-
  Add5 : Sum  Inputs=--
  Angle Conversion{4..7} (4 alike) : aerolibconvert2/Angle Conversion  IU=deg  OU=rad
  Bus Selector1 : BusSelector  OutputSignals=TVC_rY_pitch_deg,TVC_rZ_yaw_deg,TVC_lY_pitch_deg,TVC_lZ_yaw_deg
  Constant1 : Constant  Value=-1
  Constant2 : Constant  Value=-1
  Cos{2..5} (4 alike) : Trigonometry  Operator=cos
  Mux2 : Mux  Inputs=6
  Product3 : Product  Inputs=3
  Product4 : Product  Inputs=3
  Product5 : Product
  Product6 : Product
  Product7 : Product  Inputs=4
  Product8 : Product  Inputs=4
  Sin{2..5} (4 alike) : Trigonometry
  pitch1 : Product
  pitch2 : Product
  roll1 : Product
  roll2 : Product
  yaw1 : Product
  yaw2 : Product
  FM : Outport  VectorParamsAs1DForOutWhenUnconnected=off
  Tx : Outport  Port=2  VectorParamsAs1DForOutWhenUnconnected=off
  Ty : Outport  Port=3  VectorParamsAs1DForOutWhenUnconnected=off
  Tz : Outport  Port=4  VectorParamsAs1DForOutWhenUnconnected=off
  wires:
  Add5/1 -> Mux2/6  "Mz"
  Cos2/1 -> Product3/2
  Product3/1 -> Add/1  "Trx"
  Cos3/1 -> Product7/2, Product3/3
  Angle Conversion5/1 -> Cos3/1, Sin3/1
  Angle Conversion4/1 -> Cos2/1, Sin2/1
  Actuator (deg)/1 -> Bus Selector1/1
  Bus Selector1/2 -> Angle Conversion5/1  "<TVC_rZ_yaw_deg>"
  T1/1 -> Product3/1, Product4/1, Product5/1, Product6/1, Product7/1, Product8/1  "T/2"
  Mux2/1 -> FM/1
  Bus Selector1/3 -> Angle Conversion6/1  "<TVC_lY_pitch_deg>"
  Bus Selector1/4 -> Angle Conversion7/1  "<TVC_lZ_yaw_deg>"
  Bus Selector1/1 -> Angle Conversion4/1  "<TVC_rY_pitch_deg>"
  Angle Conversion6/1 -> Cos4/1, Sin4/1
  Angle Conversion7/1 -> Sin5/1, Cos5/1
  Cos4/1 -> Product4/2
  Product4/1 -> Add/2  "Tlx"
  Cos5/1 -> Product8/2, Product4/3
  Add/1 -> Mux2/1, Tx/1  "axial thrust Tx"
  Sin3/1 -> Product5/2
  Sin5/1 -> Product6/2
  Product5/1 -> yaw1/1, Add1/1  "Try"
  Product6/1 -> Add1/2, yaw2/1  "Tly"
  Add1/1 -> Mux2/2, Ty/1  "yawing thrust Ty"
  Sin2/1 -> Product7/3
  Constant1/1 -> Product7/4
  Product7/1 -> roll1/1, pitch1/1, Add2/1  "Trz"
  Sin4/1 -> Product8/3
  Constant2/1 -> Product8/4
  Product8/1 -> pitch2/1, roll2/1, Add2/2  "Tlz"
  Add2/1 -> Tz/1, Mux2/3  "pitching thrust Tz"
  " mt"/1 -> roll2/2, roll1/2  "mt"
  roll1/1 -> Add3/1
  roll2/1 -> Add3/2
  Add3/1 -> Mux2/4  "Mx"
  " lt1"/1 -> yaw2/2, yaw1/2, pitch2/2, pitch1/2  "lt1"
  pitch1/1 -> Add4/1
  pitch2/1 -> Add4/2
  Add4/1 -> Mux2/5  "My"
  yaw1/1 -> Add5/1
  yaw2/1 -> Add5/2

== system Linearize_Bare_Airframe/Vehicle/Propulsion(two_nozzles)/Actuators ==
  In Bus Element : Inport  PortName=Commands  Element=TVC_ry
  In Bus Element1 : Inport  PortName=Commands  Element=TVC_rz
  Gain4 : Gain  Gain=20.202  SaturateOnIntegerOverflow=on  OutDataTypeStr=Inherit: Same as input  ParamDataTypeStr=Inherit: Same as input
  Gain5 : Gain  Gain=20.202  SaturateOnIntegerOverflow=on  OutDataTypeStr=Inherit: Same as input  ParamDataTypeStr=Inherit: Same as input
  Rate Saturation4 : Saturate  UpperLimit=Aactuator.TVC_ry.RateLimitUpper  LowerLimit=Aactuator.TVC_ry.RateLimitLower
  Rate Saturation5 : Saturate  UpperLimit=Aactuator.TVC_rz.RateLimitUpper  LowerLimit=Aactuator.TVC_rz.RateLimitLower
  Sum4 : Sum  Inputs=|+-  InputSameDT=on  SaturateOnIntegerOverflow=on  OutDataTypeStr=Inherit: Same as first input
  Sum5 : Sum  Inputs=|+-  InputSameDT=on  SaturateOnIntegerOverflow=on  OutDataTypeStr=Inherit: Same as first input
  TVC_ry_AngleLimit : Saturate  UpperLimit=Aactuator.TVC_ry.AngleLimitUpper  LowerLimit=Aactuator.TVC_ry.AngleLimitLower
  TVC_ry_Integrator (degrees) : Integrator  InitialCondition=Aactuator.TVC_ry.IntegratorInitial  LimitOutput=on  UpperSaturationLimit=Aactuator.TVC_ry.AngleLimitUpper  LowerSaturationLimit=Aactuator.TVC_ry.AngleLimitLower
  TVC_rz_AngleLimit : Saturate  UpperLimit=Aactuator.TVC_rz.AngleLimitUpper  LowerLimit=Aactuator.TVC_rz.AngleLimitLower
  TVC_rz_Integrator (degrees) : Integrator  InitialCondition=Aactuator.TVC_rz.IntegratorInitial  LimitOutput=on  UpperSaturationLimit=Aactuator.TVC_rz.AngleLimitUpper  LowerSaturationLimit=Aactuator.TVC_rz.AngleLimitLower
  Out Bus Element : Outport  PortName=ActPositions  Element=TVC_ry_pitch_deg
  Out Bus Element1 : Outport  PortName=ActPositions  Element=TVC_rz_yaw_deg
  ActSensor_Out.TVC_ry_pitch_deg : Outport  Port=2
  ActSensor_Out.TVC_rz_yaw_deg : Outport  Port=3
  wires:
  Sum5/1 -> Gain5/1
  TVC_ry_Integrator (degrees)/1 -> Out Bus Element/1, ActSensor_Out.TVC_ry_pitch_deg/1, Sum4/2
  Sum4/1 -> Gain4/1
  In Bus Element1/1 -> TVC_rz_AngleLimit/1  "Commands_TVC_rz_yaw_deg"
  TVC_rz_Integrator (degrees)/1 -> ActSensor_Out.TVC_rz_yaw_deg/1, Out Bus Element1/1, Sum5/2
  In Bus Element/1 -> TVC_ry_AngleLimit/1  "Commands_TVC_ry_pitch_deg"
  Rate Saturation5/1 -> TVC_rz_Integrator (degrees)/1
  Gain4/1 -> Rate Saturation4/1
  Gain5/1 -> Rate Saturation5/1
  Rate Saturation4/1 -> TVC_ry_Integrator (degrees)/1
  TVC_ry_AngleLimit/1 -> Sum4/1
  TVC_rz_AngleLimit/1 -> Sum5/1

== system Linearize_Bare_Airframe/Vehicle/Propulsion(two_nozzles)/Actuators1 ==
  In Bus Element4 : Inport  PortName=Commands  Element=TVC_ly
  In Bus Element2 : Inport  PortName=Commands  Element=TVC_lz
  Gain1 : Gain  Gain=20.202  SaturateOnIntegerOverflow=on  OutDataTypeStr=Inherit: Same as input  ParamDataTypeStr=Inherit: Same as input
  Gain2 : Gain  Gain=20.202  SaturateOnIntegerOverflow=on  OutDataTypeStr=Inherit: Same as input  ParamDataTypeStr=Inherit: Same as input
  Rate Saturation1 : Saturate  UpperLimit=Aactuator.TVC_ly.RateLimitUpper  LowerLimit=Aactuator.TVC_ly.RateLimitLower
  Rate Saturation2 : Saturate  UpperLimit=Aactuator.TVC_lz.RateLimitUpper  LowerLimit=Aactuator.TVC_lz.RateLimitLower
  Sum1 : Sum  Inputs=|+-  InputSameDT=on  SaturateOnIntegerOverflow=on  OutDataTypeStr=Inherit: Same as first input
  Sum2 : Sum  Inputs=|+-  InputSameDT=on  SaturateOnIntegerOverflow=on  OutDataTypeStr=Inherit: Same as first input
  TVC_ly_AngleLimit : Saturate  UpperLimit=Aactuator.TVC_ly.AngleLimitUpper  LowerLimit=Aactuator.TVC_ly.AngleLimitLower
  TVC_ly_Integrator (degrees) : Integrator  InitialCondition=Aactuator.TVC_ly.IntegratorInitial  LimitOutput=on  UpperSaturationLimit=Aactuator.TVC_ly.AngleLimitUpper  LowerSaturationLimit=Aactuator.TVC_ly.AngleLimitLower
  TVC_lz_AngleLimit : Saturate  UpperLimit=Aactuator.TVC_lz.AngleLimitUpper  LowerLimit=Aactuator.TVC_lz.AngleLimitLower
  TVC_lz_Integrator (degrees) : Integrator  InitialCondition=Aactuator.TVC_lz.IntegratorInitial  LimitOutput=on  UpperSaturationLimit=Aactuator.TVC_lz.AngleLimitUpper  LowerSaturationLimit=Aactuator.TVC_lz.AngleLimitLower
  Out Bus Element4 : Outport  PortName=ActPositions  Element=TVC_ly_pitch_deg
  Out Bus Element5 : Outport  PortName=ActPositions  Element=TVC_lz_yaw_deg
  ActSensor_Out.TVC_ly_pitch_deg : Outport  Port=2
  ActSensor_Out.TVC_lz_yaw_deg : Outport  Port=3
  wires:
  TVC_lz_Integrator (degrees)/1 -> ActSensor_Out.TVC_lz_yaw_deg/1, Out Bus Element5/1, Sum2/2
  Gain1/1 -> Rate Saturation1/1
  Gain2/1 -> Rate Saturation2/1
  Rate Saturation1/1 -> TVC_ly_Integrator (degrees)/1
  Rate Saturation2/1 -> TVC_lz_Integrator (degrees)/1
  Sum1/1 -> Gain1/1
  In Bus Element2/1 -> TVC_lz_AngleLimit/1  "Commands_TVC_lz_yaw_deg"
  Sum2/1 -> Gain2/1
  In Bus Element4/1 -> TVC_ly_AngleLimit/1  "Commands_TVC_ly_pitch_deg"
  TVC_ly_Integrator (degrees)/1 -> ActSensor_Out.TVC_ly_pitch_deg/1, Out Bus Element4/1, Sum1/2
  TVC_ly_AngleLimit/1 -> Sum1/1
  TVC_lz_AngleLimit/1 -> Sum2/1

== system Linearize_Bare_Airframe/Vehicle/Propulsion(two_nozzles)/Afterburning Turbofan Jet Engine ==
  note: TODO: 發動機模型不完整，要看參考文獻進行更完整建模
  note: 參考文獻： Nguyen, T. Luat, et al., "Simulator Study of StallPost-Stall Characteristics of a Fighter Airplane with Relaxed Longitudinal Static Stability," NASA Technical Paper 1538 , Dec. 1979.
  note: $pow{\left(\delta_{th} \right)}={\left\{\begin{array}{c} 64.94\delta_{th} \ ,\\ 217.38\delta_{th} -117.38\ ,\ \ \ \end{array}\begin{array}{c} if{\mathrm{\ }\delta }_{th} \le 0.77\\ if{\mathrm{\ }\delta }_{th} >0.77 \end{array}\right)}$
  note: $T={\left\{\begin{array}{c} T_{idle} +{\left(T_{mil} -T_{idle} \right)}{\left(\frac{pow}{50}\right)},\ \ \ \ \ \ \ \ if\ pow<50\\ T_{mil} +{\left(T_{max} -T_{mil} \right)}{\left(\frac{pow-50}{50}\right)},\ \ \ if\ pow\ge 50 \end{array}\begin{array}{c} \ \\ \ \ \end{array}\right)}$
  note: 功率位準 power level
  note: 油門推桿位置 $0\le \delta_{th} \le 1$
  Mach : Inport
  H (ft) : Inport  Port=2
  Tc (lbf) : Inport  Port=3
  Add : Sum  Inputs=+-
  Add1 : Sum
  Add2 : Sum
  Constant : Constant
  Constant1 : Constant  Value=0
  Gain : Gain  Gain=64.94
  Gain1 : Gain  Gain=217.38
  If : If  IfExpression=u1<50  ElseIfExpressions=u1>=50  ShowElse=off
  If Action Subsystem : Subsystem  TreatAsAtomicUnit=on
  If Action Subsystem1 : Subsystem  TreatAsAtomicUnit=on
  If Action Subsystem2 : Subsystem  TreatAsAtomicUnit=on
  If Action Subsystem3 : Subsystem  TreatAsAtomicUnit=on
  If Action Subsystem4 : Subsystem  TreatAsAtomicUnit=on
  If Action Subsystem5 : Subsystem  TreatAsAtomicUnit=on
  If Action Subsystem6 : Subsystem  TreatAsAtomicUnit=on
  If1 : If  IfExpression=u1<50  ElseIfExpressions=u1>=50  ShowElse=off
  If2 : If  NumInputs=3  IfExpression=u3 == u1  ElseIfExpressions=u3>u1 & u3<=u2
  Merge : Merge  Inputs=3
  Mux : Mux  Inputs=2
  Mux1 : Mux  Inputs=2
  Mux4 : Mux  Inputs=5
  Saturation Dynamic : simulink/Discontinuities/Saturation Dynamic  OutMin=[]  OutMax=[]  OutDataTypeStr=Inherit: Same as second input  OutDataType=fixdt(1, 16)  OutScaling=2^-10  DoSatur=off
  Thrust Tidle : Interpolation_n-D  Table=EngineTable.idle  InternalRulePriority=Speed
  Thrust Tmax : Interpolation_n-D  Table=EngineTable.maximum  InternalRulePriority=Speed
  Thrust Tmil : Interpolation_n-D  Table=EngineTable.military  InternalRulePriority=Speed
  To Workspace : ToWorkspace  VariableName=T_max_min  SaveFormat=Timeseries  SampleTime=-1
  To Workspace1 : ToWorkspace  VariableName=check_engine  SaveFormat=Timeseries  SampleTime=-1
  To Workspace2 : ToWorkspace  VariableName=Mach_alt_input  SaveFormat=Timeseries  SampleTime=-1
  afterburner_off : Constant  Value=2
  afterburner_on : Constant  Value=3
  attitude Prelookup : PreLookup  BreakpointsData=EngineTable.attitude_Prelookup  IndexSearchMethod=Linear search  BeginIndexSearchUsingPreviousIndexResult=on  DiagnosticForOutOfRangeInput=Warning
  constant : Constant  Value=117.38
  idle : Constant
  mach Prelookup : PreLookup  BreakpointsData=EngineTable.mach_Prelookup  IndexSearchMethod=Linear search  BeginIndexSearchUsingPreviousIndexResult=on  DiagnosticForOutOfRangeInput=Warning
  T (lbf) : Outport  VectorParamsAs1DForOutWhenUnconnected=off
  engine_state : Outport  Port=2  VectorParamsAs1DForOutWhenUnconnected=off
  wires:
  Mach/1 -> mach Prelookup/1, Mux/2
  H (ft)/1 -> attitude Prelookup/1, Mux/1
  Add2/1 -> Saturation Dynamic/3, Mux1/2  "T_min"
  Add1/1 -> Saturation Dynamic/1, Mux1/1  "T_max"
  attitude Prelookup/2 -> Thrust Tmil/4, Thrust Tmax/4, Thrust Tidle/4
  Mux1/1 -> To Workspace/1
  Mux/1 -> To Workspace2/1
  Gain1/1 -> Add/1
  If Action Subsystem1/1(T_max1) -> Add1/2
  Constant/1 -> Gain1/1
  mach Prelookup/1 -> Thrust Tmil/1, Thrust Tmax/1, Thrust Tidle/1
  If/2 -> If Action Subsystem1/Action
  If1/2 -> If Action Subsystem3/Action
  If Action Subsystem3/1(T_min) -> Add2/2
  If Action Subsystem2/1(T_min) -> Add2/1
  If1/1 -> If Action Subsystem2/Action
  Gain/1 -> Mux4/2, If1/1  "pow"
  If Action Subsystem/1(T_max1) -> Add1/1
  mach Prelookup/2 -> Thrust Tmil/2, Thrust Tmax/2, Thrust Tidle/2
  Thrust Tidle/1 -> Mux4/3, If2/1  "Tidle"
  If/1 -> If Action Subsystem/Action
  Add/1 -> Mux4/1, If/1  "pow"
  constant/1 -> Add/2
  Mux4/1 -> If Action Subsystem1/1("input "), If Action Subsystem2/1("input "), If Action Subsystem3/1("input "), To Workspace1/1, If Action Subsystem/1("input ")
  Constant1/1 -> Gain/1
  attitude Prelookup/1 -> Thrust Tmil/3, Thrust Tmax/3, Thrust Tidle/3
  If2/1 -> If Action Subsystem4/Action
  If2/3 -> If Action Subsystem6/Action
  idle/1 -> If Action Subsystem4/1(In1)
  afterburner_on/1 -> If Action Subsystem6/1(In1)
  Thrust Tmil/1 -> If2/2, Mux4/4  "Tmil"
  Thrust Tmax/1 -> Mux4/5
  If Action Subsystem6/1(Out1) -> Merge/3
  If Action Subsystem5/1(Out1) -> Merge/2
  If Action Subsystem4/1(Out1) -> Merge/1
  afterburner_off/1 -> If Action Subsystem5/1(In1)
  If2/2 -> If Action Subsystem5/Action
  Saturation Dynamic/1 -> T (lbf)/1, If2/3  "Thrust (lbf)"
  Merge/1 -> engine_state/1
  Tc (lbf)/1 -> Saturation Dynamic/2

== system Linearize_Bare_Airframe/Vehicle/Propulsion(two_nozzles)/Thrust Vector Nozzle ZY1 ==
  note: ${\left[\begin{array}{c} F_x^{{\left(T\right)}} \\ F_y^{{\left(T\right)}} \\ F_z^{{\left(T\right)}} \end{array}\right]}={\left[\begin{array}{c} T_x \\ T_y \\ T_z \end{array}\right]}={\left[\begin{array}{c} T_{lx} \\ T_{ly} \\ T_{lz} \end{array}\right]}+{\left[\begin{array}{c} T_{rx} \\ T_{ry} \\ T_{rz} \end{array}\right]}=\frac{T}{2}{\left[\begin{array}{cc} & \cos \delta_{lz} \cos \delta_{ly} +\mathrm{cos}\delta_{rz} \cos \delta_{ry} \\ & \sin \delta_{lz} +\sin \delta_{rz} \\ - & \cos \delta_{lz} \sin \delta_{ly} -\cos \delta_{rz} \sin \delta_{ry} \end{array}\right]}$
  note: ${\left[\begin{array}{c} M_x^{{\left(T\right)}} \\ M_y^{{\left(T\right)}} \\ M_z^{{\left(T\right)}} \end{array}\right]}={\left[\begin{array}{c} M_{lx} \\ M_{ly} \\ M_{lz} \end{array}\right]}+{\left[\begin{array}{c} M_{rx} \\ M_{ry} \\ M_{rz} \end{array}\right]}=\frac{T}{2}{\left[\begin{array}{l} m_T \cos \delta_{lz} \sin \delta_{ly} -m_T \mathrm{cos}\delta_{rz} \sin \delta_{ry} \\ -l_T \cos \delta_{lz} \sin \delta_{ly} -l_T \mathrm{cos}\delta_{rz} \sin \delta_{ry} \\ {-l}_T \sin \delta_{lz} -l_T \sin \delta_{rz} \end{array}\right]}$
  note: 單一噴嘴的推力
  T1 : Inport
  Actuator (deg) : Inport  Port=2
  " lt1" : Inport  Port=3
  " mt" : Inport  Port=4
  Angle Conversion4 : aerolibconvert2/Angle Conversion  IU=deg  OU=rad
  Angle Conversion5 : aerolibconvert2/Angle Conversion  IU=deg  OU=rad
  Bus Selector1 : BusSelector  OutputSignals=TVC_ry_pitch_deg,TVC_rz_yaw_deg
  Constant1 : Constant  Value=-1
  Constant2 : Constant  Value=-1
  Cos2 : Trigonometry  Operator=cos
  Cos3 : Trigonometry  Operator=cos
  Product3 : Product  Inputs=3
  Product5 : Product
  Product7 : Product  Inputs=4
  Sin2 : Trigonometry
  Sin3 : Trigonometry
  pitch1 : Product
  roll1 : Product
  yaw1 : Product  Inputs=3
  Trx : Outport  VectorParamsAs1DForOutWhenUnconnected=off
  Try : Outport  Port=2  VectorParamsAs1DForOutWhenUnconnected=off
  Trz : Outport  Port=3  VectorParamsAs1DForOutWhenUnconnected=off
  Mrx : Outport  Port=4  VectorParamsAs1DForOutWhenUnconnected=off
  Mry : Outport  Port=5  VectorParamsAs1DForOutWhenUnconnected=off
  Mrz : Outport  Port=6  VectorParamsAs1DForOutWhenUnconnected=off
  wires:
  yaw1/1 -> Mrz/1  "Mrz"
  Cos2/1 -> Product3/2
  Product3/1 -> Trx/1  "Trx"
  Cos3/1 -> Product7/2, Product3/3
  Angle Conversion5/1 -> Cos3/1, Sin3/1
  Angle Conversion4/1 -> Cos2/1, Sin2/1
  Actuator (deg)/1 -> Bus Selector1/1
  Bus Selector1/2 -> Angle Conversion5/1  "<TVC_rz_yaw_deg>"
  T1/1 -> Product3/1, Product5/1, Product7/1  "T/2"
  Bus Selector1/1 -> Angle Conversion4/1  "<TVC_ry_pitch_deg>"
  Sin3/1 -> Product5/2
  Product5/1 -> Try/1, yaw1/1  "Try"
  Sin2/1 -> Product7/3
  Constant1/1 -> Product7/4
  Product7/1 -> roll1/1, pitch1/1, Trz/1  "Trz"
  " mt"/1 -> roll1/2  "mt"
  roll1/1 -> Mrx/1  "Mrx"
  " lt1"/1 -> yaw1/2, pitch1/2  "lt1"
  pitch1/1 -> Mry/1  "Mry"
  Constant2/1 -> yaw1/3

== system Linearize_Bare_Airframe/Vehicle/Propulsion(two_nozzles)/Thrust Vector Nozzle ZY2 ==
  note: ${\left[\begin{array}{c} F_x^{{\left(T\right)}} \\ F_y^{{\left(T\right)}} \\ F_z^{{\left(T\right)}} \end{array}\right]}={\left[\begin{array}{c} T_x \\ T_y \\ T_z \end{array}\right]}={\left[\begin{array}{c} T_{lx} \\ T_{ly} \\ T_{lz} \end{array}\right]}+{\left[\begin{array}{c} T_{rx} \\ T_{ry} \\ T_{rz} \end{array}\right]}=\frac{T}{2}{\left[\begin{array}{cc} & \cos \delta_{lz} \cos \delta_{ly} +\mathrm{cos}\delta_{rz} \cos \delta_{ry} \\ & \sin \delta_{lz} +\sin \delta_{rz} \\ - & \cos \delta_{lz} \sin \delta_{ly} -\cos \delta_{rz} \sin \delta_{ry} \end{array}\right]}$
  note: ${\left[\begin{array}{c} M_x^{{\left(T\right)}} \\ M_y^{{\left(T\right)}} \\ M_z^{{\left(T\right)}} \end{array}\right]}={\left[\begin{array}{c} M_{lx} \\ M_{ly} \\ M_{lz} \end{array}\right]}+{\left[\begin{array}{c} M_{rx} \\ M_{ry} \\ M_{rz} \end{array}\right]}=\frac{T}{2}{\left[\begin{array}{l} m_T \cos \delta_{lz} \sin \delta_{ly} -m_T \mathrm{cos}\delta_{rz} \sin \delta_{ry} \\ -l_T \cos \delta_{lz} \sin \delta_{ly} -l_T \mathrm{cos}\delta_{rz} \sin \delta_{ry} \\ {-l}_T \sin \delta_{lz} -l_T \sin \delta_{rz} \end{array}\right]}$
  note: 單一噴嘴的推力
  T1 : Inport
  Actuator (deg) : Inport  Port=2
  " lt1" : Inport  Port=3
  " mt" : Inport  Port=4
  Angle Conversion6 : aerolibconvert2/Angle Conversion  IU=deg  OU=rad
  Angle Conversion7 : aerolibconvert2/Angle Conversion  IU=deg  OU=rad
  Bus Selector1 : BusSelector  OutputSignals=TVC_ly_pitch_deg,TVC_lz_yaw_deg
  Constant1 : Constant  Value=-1
  Constant2 : Constant  Value=-1
  Constant3 : Constant  Value=-1
  Cos4 : Trigonometry  Operator=cos
  Cos5 : Trigonometry  Operator=cos
  Product4 : Product  Inputs=3
  Product6 : Product
  Product8 : Product  Inputs=4
  Sin4 : Trigonometry
  Sin5 : Trigonometry
  pitch2 : Product
  roll2 : Product  Inputs=3
  yaw2 : Product  Inputs=3
  Tlx : Outport  VectorParamsAs1DForOutWhenUnconnected=off
  Tly : Outport  Port=2  VectorParamsAs1DForOutWhenUnconnected=off
  Tlz : Outport  Port=3  VectorParamsAs1DForOutWhenUnconnected=off
  Mlx : Outport  Port=4  VectorParamsAs1DForOutWhenUnconnected=off
  Mly : Outport  Port=5  VectorParamsAs1DForOutWhenUnconnected=off
  Mlz : Outport  Port=6  VectorParamsAs1DForOutWhenUnconnected=off
  wires:
  yaw2/1 -> Mlz/1  "Mlz"
  Actuator (deg)/1 -> Bus Selector1/1
  T1/1 -> Product4/1, Product8/1, Product6/1  "T/2"
  Bus Selector1/1 -> Angle Conversion6/1  "<TVC_ly_pitch_deg>"
  Bus Selector1/2 -> Angle Conversion7/1  "<TVC_lz_yaw_deg>"
  Angle Conversion6/1 -> Cos4/1, Sin4/1
  Angle Conversion7/1 -> Sin5/1, Cos5/1
  Cos4/1 -> Product4/2
  Product4/1 -> Tlx/1  "Tlx"
  Cos5/1 -> Product8/2, Product4/3
  Sin5/1 -> Product6/2
  Product6/1 -> yaw2/1, Tly/1  "Tly"
  Sin4/1 -> Product8/3
  Constant2/1 -> Product8/4
  Product8/1 -> pitch2/1, roll2/1, Tlz/1  "Tlz"
  " mt"/1 -> roll2/2  "mt"
  roll2/1 -> Mlx/1  "Mlx"
  " lt1"/1 -> yaw2/2, pitch2/2  "lt1"
  pitch2/1 -> Mly/1  "Mly"
  Constant1/1 -> roll2/3
  Constant3/1 -> yaw2/3
